simulink model "testNserver_SimEvents"  (R2023a)
settings: Solver=VariableStepAuto  StartTime=0.0  StopTime=10.0  RelTol=1e-3
InitFcn:
  | tG = 1.0;  % intergeneration time
  | tS = 2.8;  % service time
  | N = 6;    % total number of entities to create
undefined symbols (not defined in the file or in its folder): entity, m, n, showValue
settings Model: Creator=peter  LastModifiedBy=peter

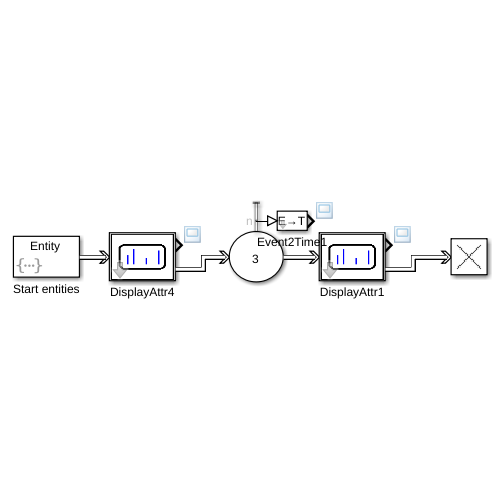
[thumbnail: Simulink's stored preview of the top-level diagram]
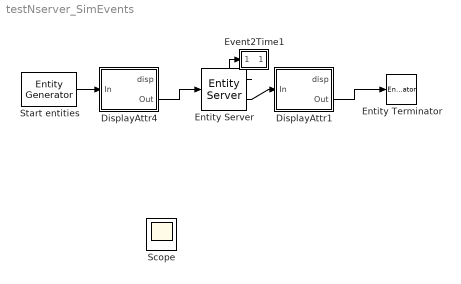
== system testNserver_SimEvents ==
  DisplayAttr1 : Subsystem  mask(DisplayId){w=0.001, attrib=id}
      mask prompts: w "Signal width"; attrib "Attribute"
      mask help: Provides a port to display an attribute of passing entities.
      mask init:
      | varName = ['entity.', strtrim(attrib)];
      | block = [gcb, '/EntityServer'];
      | set_param(block, 'PostArrivalFunction', ['showValue(' varName ');']);
      mask Display: image('$imagefile'); % Use "Edit Image" on toolstrip to change.
  DisplayAttr4 : Subsystem  mask(DisplayId){w=0.001, attrib=id}
      mask prompts: w "Signal width"; attrib "Attribute"
      mask help: Provides a port to display an attribute of passing entities.
      mask init:
      | varName = ['entity.', strtrim(attrib)];
      | block = [gcb, '/EntityServer'];
      | set_param(block, 'PostArrivalFunction', ['showValue(' varName ');']);
      mask Display: image('$imagefile'); % Use "Edit Image" on toolstrip to change.
  Entity Server : EntityServer  InputPortMessageModes=m  OutputPortMessageModes=n,m  Capacity=3  ServiceTimeSource=MATLAB action  ServiceTimeValue=1  ServiceTimeAction=dt = tS;  NumberEntitiesInBlock=on
      settings: OutputPortMap=o1,o9
  Entity Terminator : EntityTerminator  InputPortMessageModes=m
  Event2Time1 : Subsystem  mask(Event2Time){}
      mask help: Changes Signal from event-driven to time-driven.
      mask Display: disp('E→T')
  Start entities : EntityGenerator  OutputPortMessageModes=m  TimeSource=MATLAB action  IntergenerationTimeAction=|  GenerateEntityAtSimulationStart=off  GenerateAction=|  AttributeName=id  AttributeInitialValue=0  EntityType=Structured  EntityTypeName=Entity
      IntergenerationTimeAction=|
      | % create N entities in time steps of tG
      | persistent nr;
      | if isempty(nr)
      |   nr = 1;
      | end
      | if nr <= N
      |   dt = tG;
      | else
      |   dt = inf;
      | end
      | nr = nr + 1;
      GenerateAction=|
      | % set id attribut
      | persistent next_id
      | if isempty(next_id)
      |   next_id = 1;
      | end
      | 
      | entity.id = next_id;
      | next_id = next_id + 1;
  Scope : Scope
  wires:
  Start entities/1 -> DisplayAttr4/1(In)
  DisplayAttr4/2(Out) -> Entity Server/1
  DisplayAttr1/2(Out) -> Entity Terminator/1
  Entity Server/2 -> DisplayAttr1/1(In)
  Entity Server/1 -> Event2Time1/1(In1)

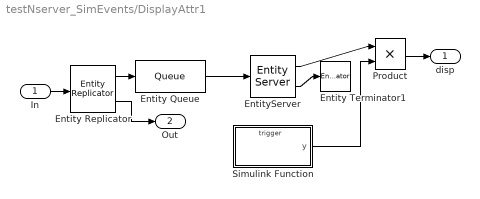
== system testNserver_SimEvents/DisplayAttr1 ==
  In : Inport
  Entity Queue : Queue  InputPortMessageModes=m  OutputPortMessageModes=m  Capacity=inf
  Entity Replicator : EntityReplicator  InputPortMessageModes=m  OutputPortMessageModes=m,m  HoldOriginalEntityUntilAllReplicasDepart=on
  Entity Terminator1 : EntityTerminator  InputPortMessageModes=m
  EntityServer : EntityServer  InputPortMessageModes=m  OutputPortMessageModes=n,m  Capacity=1  ServiceTimeValue=w  EntryAction=showValue(entity.id);  NumberEntitiesInBlock=on
      settings: OutputPortMap=o1,o9
  Product : Product
  Simulink Function : Subsystem  TreatAsAtomicUnit=on
  disp : Outport  VectorParamsAs1DForOutWhenUnconnected=off
  Out : Outport  Port=2  VectorParamsAs1DForOutWhenUnconnected=off
  wires:
  Entity Replicator/2 -> Out/1
  Entity Replicator/1 -> Entity Queue/1
  Product/1 -> disp/1
  Simulink Function/1(y) -> Product/2
  EntityServer/1 -> Product/1
  Entity Queue/1 -> EntityServer/1
  EntityServer/2 -> Entity Terminator1/1
  In/1 -> Entity Replicator/1

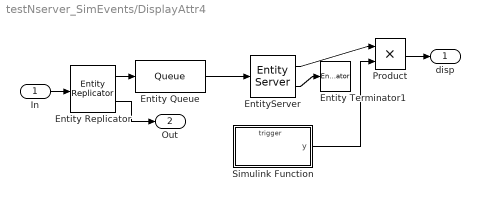
== system testNserver_SimEvents/DisplayAttr4 ==
  In : Inport
  Entity Queue : Queue  InputPortMessageModes=m  OutputPortMessageModes=m  Capacity=inf
  Entity Replicator : EntityReplicator  InputPortMessageModes=m  OutputPortMessageModes=m,m  HoldOriginalEntityUntilAllReplicasDepart=on
  Entity Terminator1 : EntityTerminator  InputPortMessageModes=m
  EntityServer : EntityServer  InputPortMessageModes=m  OutputPortMessageModes=n,m  Capacity=1  ServiceTimeValue=w  EntryAction=showValue(entity.id);  NumberEntitiesInBlock=on
      settings: OutputPortMap=o1,o9
  Product : Product
  Simulink Function : Subsystem  TreatAsAtomicUnit=on
  disp : Outport  VectorParamsAs1DForOutWhenUnconnected=off
  Out : Outport  Port=2  VectorParamsAs1DForOutWhenUnconnected=off
  wires:
  Entity Replicator/2 -> Out/1
  Entity Replicator/1 -> Entity Queue/1
  Product/1 -> disp/1
  Simulink Function/1(y) -> Product/2
  EntityServer/1 -> Product/1
  Entity Queue/1 -> EntityServer/1
  EntityServer/2 -> Entity Terminator1/1
  In/1 -> Entity Replicator/1

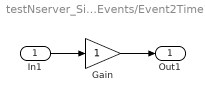
== system testNserver_SimEvents/Event2Time1 ==
  In1 : Inport
  Gain : Gain
  Out1 : Outport  VectorParamsAs1DForOutWhenUnconnected=off
  wires:
  Gain/1 -> Out1/1
  In1/1 -> Gain/1

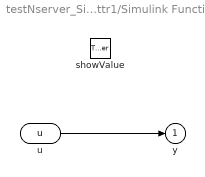
== system testNserver_SimEvents/DisplayAttr1/Simulink Function ==
  showValue : TriggerPort  TriggerType=function-call  IsSimulinkFunction=on  FunctionName=showValue  FunctionVisibility=scoped  VariantControl=Variant
  u : ArgIn  DisableCoverage=on  ArgumentName=u
  y : Outport  VectorParamsAs1DForOutWhenUnconnected=off
  wires:
  u/1 -> y/1

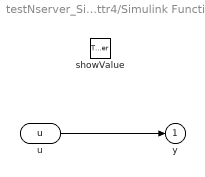
== system testNserver_SimEvents/DisplayAttr4/Simulink Function ==
  showValue : TriggerPort  TriggerType=function-call  IsSimulinkFunction=on  FunctionName=showValue  FunctionVisibility=scoped  VariantControl=Variant
  u : ArgIn  DisableCoverage=on  ArgumentName=u
  y : Outport  VectorParamsAs1DForOutWhenUnconnected=off
  wires:
  u/1 -> y/1
